simulink model "zeitdiskrete_Regelkreis"  (Simulink 9.1)
settings: Solver=VariableStepAuto  StartTime=0.0  StopTime=10  RelTol=1e-3
values from neighbouring files (symbols this model uses):
  FI = expm(A*Ta)    [main4.m]
  H = inv(A)*(FI - I)*B    [main4.m]
  Km = 1/Fn    (= 1.5873015873e-05)    [main4.m]
undefined symbols (not defined in the file or in its folder): C, D, DiscIntNeverNeededParam
settings Model: Creator=Emily  LastModifiedBy=Emily
settings DataIOCC: SaveFormat=Dataset
settings OptimizationCC: LifeSpan=auto
settings DebuggingCC: UnderspecifiedInitializationDetection=Simplified  MergeDetectMultiDrivingBlocksExec=error  SFUnexpectedBacktrackingDiag=error  SFNoUnconditionalDefaultTransitionDiag=error  SFExecutionAtInitializationDiag=warning
settings HardwareCC: ProdBitPerPointer=64  ProdBitPerSizeT=64  ProdBitPerPtrDiffT=64  ProdLargestAtomicFloat=Float  ProdIntDivRoundTo=Zero  ProdEndianess=LittleEndian  ProdWordSize=64  ProdHWDeviceType=Intel->x86-64 (Windows64)
settings ModelReferenceCC: PropagateSignalLabelsOutOfModel=on
settings CodeAppCC: StateflowObjectComments=off
settings GRTTargetCC: TargetLangStandard=C99 (ISO)  CombineOutputUpdateFcns=on  GRTInterface=off
settings ConfigComp: CovMetricSettings=dwe  CovHtmlReporting=off  CovSaveCumulativeToWorkspaceVar=off  CovSaveSingleToWorkspaceVar=off  CovExternalEMLEnable=on

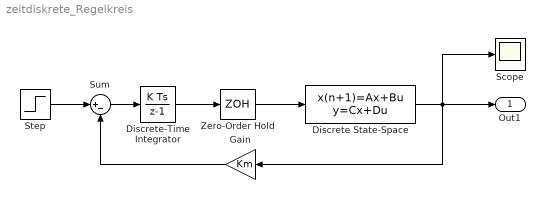
== system zeitdiskrete_Regelkreis ==
  Discrete State-Space : DiscreteStateSpace  A=FI  B=H  C=C  D=D  SampleTime=0.015
  Discrete-Time Integrator : DiscreteIntegrator  gainval=0.25  SampleTime=0.015  ICPrevOutput=DiscIntNeverNeededParam  ICPrevScaledInput=DiscIntNeverNeededParam
  Gain : Gain  Gain=Km
  Scope : Scope
  Step : Step  After=0.8  SampleTime=0
  Sum : Sum  Inputs=|+-
  Zero-Order Hold : ZeroOrderHold  SampleTime=0.015
  Out1 : Outport
  wires:
  Discrete-Time Integrator/1 -> Zero-Order Hold/1
  Zero-Order Hold/1 -> Discrete State-Space/1
  Sum/1 -> Discrete-Time Integrator/1
  Gain/1 -> Sum/2
  Discrete State-Space/1 -> Out1/1, Gain/1, Scope/1
  Step/1 -> Sum/1
